simulink model "robot_sim_TamePID_separated"  (R2025b)
settings: Solver=VariableStepAuto  StartTime=0.0  StopTime=10.0  RelTol=1e-3
values from neighbouring files (symbols this model uses):
  alpha = 1    [FIREFIGHTER_AID.m]    (also in Setup_CSDR_Simulation.m = -1.57079632679; Setup_CSDR_Simulation_NL.m = -1.57079632679)
  D = [d1 0; 0 d2]    [Setup_CSDR_Simulation.m]    (also in Setup_CSDR_Simulation_NL.m)
  g = 1    [FIREFIGHTER_AID.m]    (also in Setup_CSDR_Simulation.m = 9.81; Setup_CSDR_Simulation_NL.m = 9.81)
  I1 = 1.5    [Setup_CSDR_Simulation.m]    (also in Setup_CSDR_Simulation_NL.m)
  I2 = 0.5    [Setup_CSDR_Simulation.m]    (also in Setup_CSDR_Simulation_NL.m)
  Kd1 = 250    [Setup_CSDR_Simulation.m]
  Kd2 = 150    [Setup_CSDR_Simulation.m]
  Ki1 = 150    [Setup_CSDR_Simulation.m]
  Ki2 = 120    [Setup_CSDR_Simulation.m]
  Kp1 = 500    [Setup_CSDR_Simulation.m]
  Kp2 = 400    [Setup_CSDR_Simulation.m]
  l_c1 = 1    [FIREFIGHTER_AID.m]    (also in Setup_CSDR_Simulation.m = 0.5; Setup_CSDR_Simulation_NL.m = 0.5)
  m1 = 1    [FIREFIGHTER_AID.m]    (also in Setup_CSDR_Simulation.m = 15; Setup_CSDR_Simulation_NL.m = 15)
  m2 = 1    [FIREFIGHTER_AID.m]    (also in Setup_CSDR_Simulation.m = 8; Setup_CSDR_Simulation_NL.m = 8)
  S = eye(2)    [Setup_CSDR_Simulation.m]    (also in Setup_CSDR_Simulation_NL.m)
settings Model: Creator=sjoer  LastModifiedBy=Ricardo Díaz

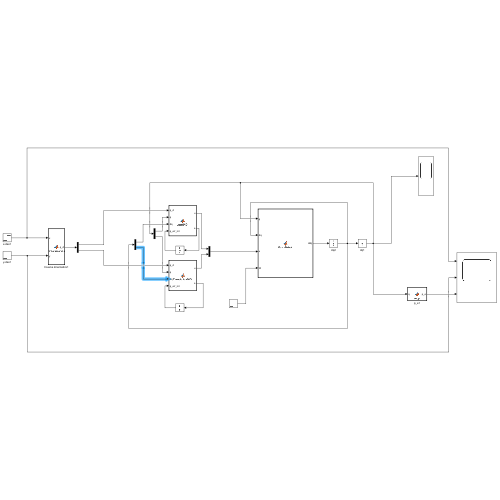
[thumbnail: Simulink's stored preview of the top-level diagram]
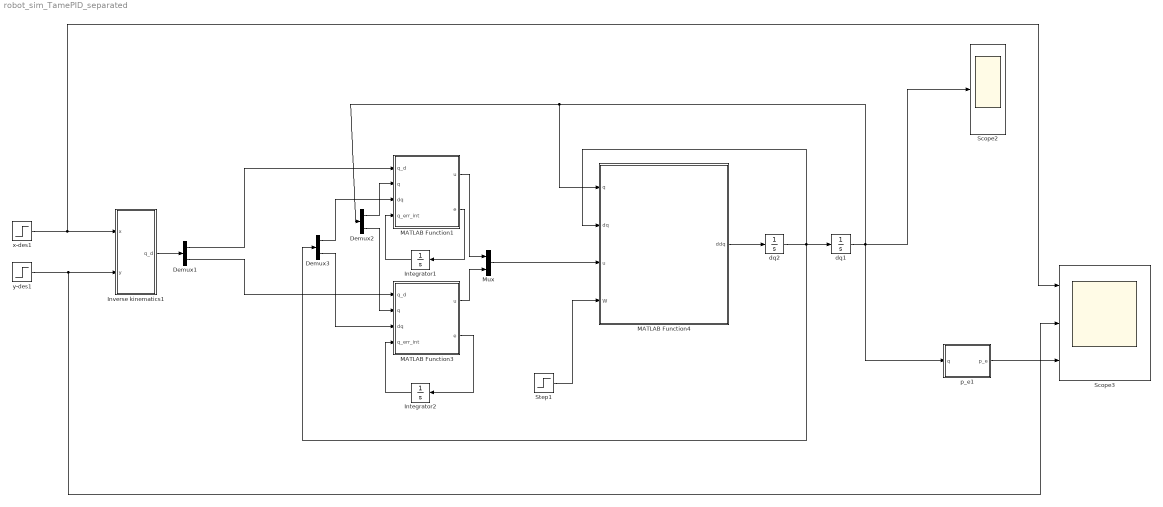
== system robot_sim_TamePID_separated ==
  Demux1 : Demux  Outputs=2
  Demux2 : Demux  Outputs=2
  Demux3 : Demux  Outputs=2
  Integrator1 : Integrator
  Integrator2 : Integrator
  Inverse kinematics1 : MATLAB Function  TreatAsAtomicUnit=on
  MATLAB Function1 : MATLAB Function  TreatAsAtomicUnit=on
  MATLAB Function3 : MATLAB Function  TreatAsAtomicUnit=on
  MATLAB Function4 : MATLAB Function  TreatAsAtomicUnit=on
  Mux : Mux  Inputs=2
  Scope2 : Scope
      settings: ActiveDisplayYMinimum=-1.4051776468584192  ActiveDisplayYMaximum=7.2505527137627759  DataLoggingVariableName=ScopeData2
  Scope3 : Scope  NumInputPorts=3
      settings: ActiveDisplayYMinimum=-3.1931874410445822  ActiveDisplayYMaximum=4.9083084167084117  DataLoggingVariableName=ScopeData3
  Step1 : Step  After=[0;0]  SampleTime=0
  dq1 : Integrator
  dq2 : Integrator
  p_e1 : MATLAB Function  TreatAsAtomicUnit=on
  x-des1 : Step  Time=2  After=0.5  SampleTime=0
  y-des1 : Step  Time=2  SampleTime=0
  wires:
  Inverse kinematics1/1(q_d) -> Demux1/1
  Demux1/1 -> MATLAB Function1/1(q_d)
  Demux1/2 -> MATLAB Function3/1(q_d)
  MATLAB Function4/1(ddq) -> dq2/1
  dq2/1 -> MATLAB Function4/2(dq), Demux3/1, dq1/1
  x-des1/1 -> Scope3/1, Inverse kinematics1/1(x)
  y-des1/1 -> Scope3/2, Inverse kinematics1/2(y)
  Demux2/1 -> MATLAB Function1/2(q)
  Demux2/2 -> MATLAB Function3/2(q)
  MATLAB Function1/1(u) -> Mux/1
  MATLAB Function3/1(u) -> Mux/2
  MATLAB Function1/2(e) -> Integrator1/1
  Integrator1/1 -> MATLAB Function1/4(q_err_int)
  MATLAB Function3/2(e) -> Integrator2/1
  Integrator2/1 -> MATLAB Function3/4(q_err_int)
  Demux3/1 -> MATLAB Function1/3(dq)
  Demux3/2 -> MATLAB Function3/3(dq)
  Step1/1 -> MATLAB Function4/4(W)
  dq1/1 -> MATLAB Function4/1(q), Demux2/1, Scope2/1, p_e1/1(q)
  p_e1/1(p_e) -> Scope3/3
  Mux/1 -> MATLAB Function4/3(u)

== matlab function robot_sim_TamePID_separated/MATLAB Function1 ==
  data: q_d input size=1 1; u output size=1 1; q input size=1 1; dq input size=1 1; q_err_int input size=1 1; Kp1 parameter; Ki1 parameter; Kd1 parameter; e output size=1 1
function [u,e] = JointPID(q_d, q, dq, q_err_int, Kp1, Ki1, Kd1)
% Scalar joint PID controller

% Error
e = q_d - q;


% Joint 1 (Rotation)
u = (Kp1 * e) + (Ki1 * q_err_int) - (Kd1 * dq); %tau
end

== matlab function robot_sim_TamePID_separated/MATLAB Function3 ==
  data: q_d input size=1 1; u output size=1 1; q input size=1 1; dq input size=1 1; q_err_int input size=1 1; Kp2 parameter; Ki2 parameter; Kd2 parameter; e output size=1 1
function [u,e] = TranslationPID(q_d, q, dq, q_err_int, Kp2, Ki2, Kd2)
% Scalar joint PID controller

% Error
e = q_d - q;

% Joint 2 (Prismatic)
u = (Kp2 * e) + (Ki2 * q_err_int) - (Kd2 * dq); %F
end

== matlab function robot_sim_TamePID_separated/Inverse kinematics1 ==
  data: x input; q_d output size=2 1; y input
function q_d  = InverseKinematics(x, y)
    % This block runs every time step
    
    % Extension (Prismatic Joint)
    q2_d = sqrt(x^2 + y^2);
    
    % Rotation (Revolute Joint)
    % We use atan2 to handle all quadrants automatically
    q1_d = atan2(y, x);

    q_d = [q1_d; q2_d];
end

== matlab function robot_sim_TamePID_separated/MATLAB Function4 ==
  data: q input; ddq output; dq input; u input; W input; I1 parameter; I2 parameter; l_c1 parameter; m1 parameter; m2 parameter; S parameter; D parameter; g parameter; alpha parameter
function ddq  = PolarRobot(q, dq, u, W, I1, I2, l_c1, m1, m2, S, D, g, alpha)
% Only the dynamic equations remain here

% Vectors
q1 = q(1);
q2 = q(2);
dq_1 = dq(1);
dq_2 = dq(2);

% M(q) - Mass matrix (Changes with q2)
M = [I1 + I2 + (l_c1^2)*m1 + m2*(q2^2), 0;
     0, m2];

% c(q,dq) - Coriolis (Changes with q2, dq1, dq2)
c = [2*dq_1*dq_2*m2*q2;
    -(dq_1^2)*m2*q2];

% G(q) - Gravity (Changes with q1, q2)
G = [g*cos(alpha - q1)*(l_c1*m1 + m2*q2);
    -g*m2*sin(alpha - q1)];

% J(q) - Jacobian
J = [-q2*sin(q1), cos(q1);
      q2*cos(q1), sin(q1)];

% Solving for ddq
ddq = M \ (S*u + J'* W - c - D*dq - G);

== matlab function robot_sim_TamePID_separated/p_e1 ==
  data: q input; p_e output
function p_e = ee_p(q)

p_e = [q(2)*cos(q(1)); q(2)*sin(q(1))];
